simulink model "stopforce"  (R2022b)
settings: Solver=VariableStepAuto  StartTime=0.0  StopTime=7  RelTol=1e-3
libraries: simulink x1
settings Model: Creator=giaco  LastModifiedBy=giaco

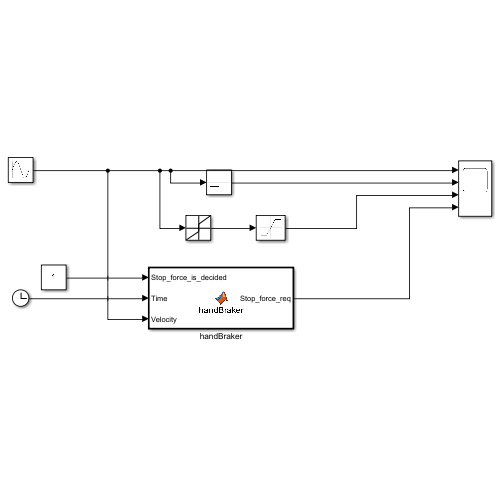
[thumbnail: Simulink's stored preview of the top-level diagram]
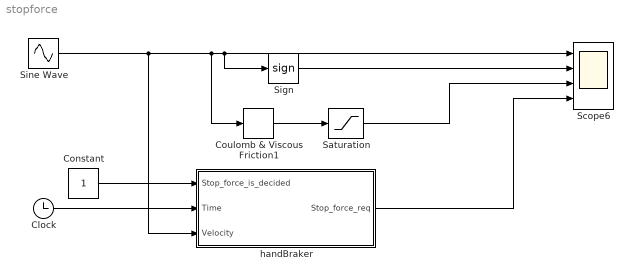
== system stopforce ==
  Clock : Clock
  Constant : Constant
  Coulomb & Viscous Friction1 : simulink/Discontinuities/Coulomb & Viscous Friction  offset=4  gain=10
  Saturation : Saturate  UpperLimit=0  LowerLimit=-Inf
  Scope6 : Scope  NumInputPorts=4
  Sign : Signum
  Sine Wave : Sin  SampleTime=0
  handBraker : MATLAB Function  TreatAsAtomicUnit=on
  wires:
  Sine Wave/1 -> handBraker/3(Velocity), Scope6/1, Sign/1, Coulomb & Viscous Friction1/1
  Coulomb & Viscous Friction1/1 -> Saturation/1
  Saturation/1 -> Scope6/3
  Sign/1 -> Scope6/2
  Constant/1 -> handBraker/1(Stop_force_is_decided)
  Clock/1 -> handBraker/2(Time)
  handBraker/1(Stop_force_req) -> Scope6/4

== matlab function stopforce/handBraker ==
  data: Stop_force_is_decided input; Time input; Velocity input; Stop_force_req output
function Stop_force_req = handBraker(Stop_force_is_decided, Time, Velocity)

Stop_force_req = 0;

if Stop_force_is_decided % || (Velocity < 0 && Time > 10)
    Stop_force_req = 10 * sign(Velocity);
end % if
